simulink model "x2Stage_Rocket"  (R2022b)
settings: Solver=VariableStepAuto  StartTime=0.0  StopTime=5
model workspace: external: MATLAB File C:\Users\Trenton VerKuilen\OneDrive - lmu.edu\School\Capstone\SimscapeImportFiles\x2Stage_Rocket_DataFile.m (data not in the file)
undefined symbols (not defined in the file or in its folder): F, MIL, Moderate, sigbuilder_block, smiData, X, Y, Z
libraries: sm_lib x543, nesl_utility x11, simulink_extras x3, sharedtransform x2, dspmtrx3 x2, aerolibwind2 x2, mspsensorlib x1, aerolibatmos2 x1
(part 1 of 11)
settings Model: Creator=Poseidon  LastModifiedBy=Poseidon
settings SolverCC: MaxConsecutiveZCs=auto  ZeroCrossAlgorithm=Adaptive
settings OptimizationCC: EnhancedBackFolding=on  PassReuseOutputArgsAs=Individual arguments  ZeroExternalMemoryAtStartup=off  ZeroInternalMemoryAtStartup=off  MaxStackSize=64  OptimizeBlockOrder=speed  DifferentSizesBufferReuse=on  EfficientTunableParamExpr=on
settings DebuggingCC: IgnoredZcDiagnostic=none  ParameterTunabilityLossMsg=error
settings SFSimCC: MATLABDynamicMemAlloc=off
settings RTWCC: Description=Embedded Coder  SystemTargetFile=ert.tlc  HardwareBoard=Robot Operating System 2 (ROS 2)  TLCOptions="-aInlineSetEventsForThisBaseRateFcn=TLC_FALSE -aSuppressMultiTaskScheduler=TLC_FALSE  -aRateBasedStepFcn=0"  TemplateMakefile=ert_default_tmf  Toolchain=Colcon Tools  TargetLang=C++
settings CodeAppCC: ForceParamTrailComments=on  IgnoreCustomStorageClasses=off  OperatorAnnotations=on  SimulinkDataObjDesc=on  SFDataObjDesc=on  InsertBlockDesc=on
settings ERTTargetCC: CodeInterfacePackaging=C++ class  RootIOFormat=Structure reference

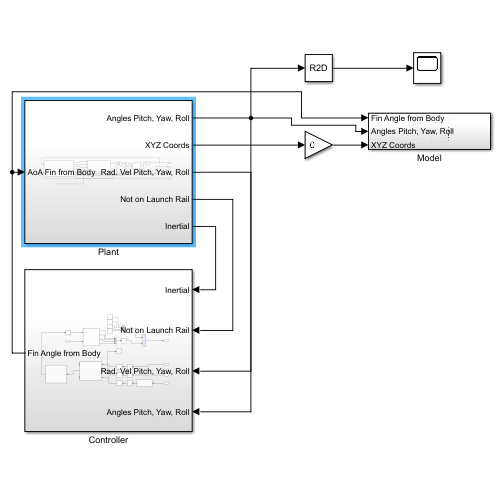
[thumbnail: Simulink's stored preview of the top-level diagram]
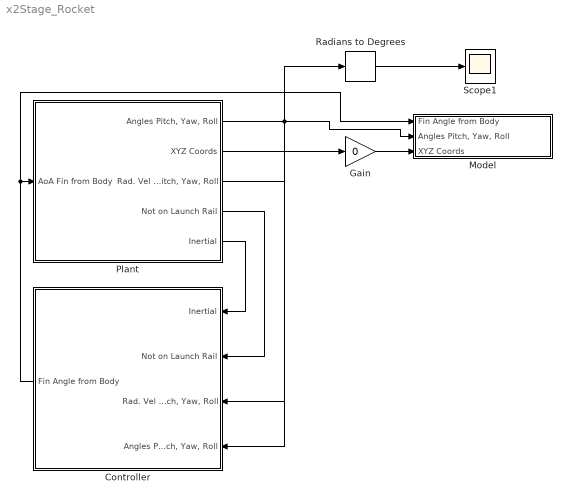
== system x2Stage_Rocket ==
  Controller : Subsystem
  Gain : Gain  Gain=0
  Model : Subsystem
  Plant : Subsystem
  Radians to Degrees : simulink_extras/Transformations/Radians to Degrees
  Scope1 : Scope
  wires:
  Radians to Degrees/1 -> Scope1/1
  Plant/3("Rad. Vel Pitch, Yaw, Roll") -> Controller/3("Rad. Vel Pitch, Yaw, Roll")
  Plant/5(Inertial) -> Controller/1(Inertial)
  Plant/4(Not on Launch Rail) -> Controller/2(Not on Launch Rail)
  Plant/2(XYZ Coords) -> Gain/1
  Gain/1 -> Model/3(XYZ Coords)
  Controller/1(Fin Angle from Body) -> Model/1(Fin Angle from Body), Plant/1(AoA Fin from Body)
  Plant/1("Angles Pitch, Yaw, Roll") -> Controller/4("Angles Pitch, Yaw, Roll"), Model/2("Angles Pitch, Yaw, Roll"), Radians to Degrees/1

== system x2Stage_Rocket/Controller ==
  Inertial : Inport
  Not on Launch Rail : Inport  Port=2
  "Rad. Vel Pitch, Yaw, Roll" : Inport  Port=3
  "Angles Pitch, Yaw, Roll" : Inport  Port=4
  Complex to Real-Imag : ComplexToRealImag  Output=Real
  Constant{,1..3} (4 alike) : Constant  Value=0
  Degrees to Radians : simulink_extras/Transformations/Degrees to Radians
  Double Click to Toggle2 : ManualSwitch  CurrentSetting=0
  MPU 6050 : mspsensorlib/IMU  DispRefFrame=NED  Temperature=25  MagneticFieldNED=[ 27.5550, -2.4169, -16.0849 ]  MagneticFieldENU=[ -2.4169, 27.5550, 16.0849 ]  SeedDouble=67  SimulateUsing=Code generation  AccelParamsMeasurementRange=160  AccelParamsResolution=0.00479  AccelParamsConstantBias=[ 0, 0, 0 ]  AccelParamsAxesMisalignment=[ 100, 0, 0; 0, 100, 0; 0, 0, 100 ]  AccelParamsNoiseDensity=[ 0, 0, 0 ]  AccelParamsBiasInstability=[ 0, 0, 0 ]  AccelParamsRandomWalk=[ 0, 0, 0 ]  AccelParamsTemperatureBias=[ 0, 0, 0 ]  AccelParamsTemperatureScaleFactor=[ 0, 0, 0 ]  GyroParamsMeasurementRange=4.36332  GyroParamsResolution=0.000133157958984  GyroParamsConstantBias=[ 0, 0, 0 ]  GyroParamsAxesMisalignment=[ 100, 0, 0; 0, 100, 0; 0, 0, 100 ]  GyroParamsAccelerationBias=[ 0, 0, 0 ]  GyroParamsNoiseDensity=[ 5.24*10^-5, 5.24*10^-5, 5.24*10^-5 ]  GyroParamsBiasInstability=[ 2.09*10^-5, 2.09*10^-5, 2.09*10^-5 ]  GyroParamsRandomWalk=[ 0, 0, 0 ]  GyroParamsTemperatureBias=[ 0, 0, 0 ]  GyroParamsTemperatureScaleFactor=[ 0, 0, 0 ]  MagParamsMeasurementRange=Inf  MagParamsResolution=0  MagParamsConstantBias=[ 0, 0, 0 ]  MagParamsAxesMisalignment=[ 100, 0, 0; 0, 100, 0; 0, 0, 100 ]  MagParamsNoiseDensity=[ 0, 0, 0 ]  MagParamsBiasInstability=[ 0, 0, 0 ]  MagParamsRandomWalk=[ 0, 0, 0 ]  MagParamsTemperatureBias=[ 0, 0, 0 ]  MagParamsTemperatureScaleFactor=[ 0, 0, 0 ]
  Mux2 : Mux
  Mux3 : Mux
  PID : Subsystem
  Rotation Angles to Quaternions : sharedtransform/Rotation Angles to Quaternions  rotationOrder=YZX  aMode=aMode
  Scope : Scope
  Transpose : Math  Operator=transpose
  Transpose1 : Math  Operator=transpose
  Transpose2 : Math  Operator=transpose
  Unscented Kalman Filter : Subsystem
  Zero-Order Hold : ZeroOrderHold  SampleTime=0.001
  Zero-Order Hold1 : ZeroOrderHold  SampleTime=0.001
  Zero-Order Hold2 : ZeroOrderHold  SampleTime=0.001
  Fin Angle from Body : Outport
  wires:
  Constant3/1 -> Mux3/4
  PID/1(Fin 1) -> Mux2/1
  Mux2/1 -> Degrees to Radians/1
  PID/4(Fin 4) -> Mux2/4
  Constant2/1 -> Mux3/3
  Constant/1 -> Mux3/1
  PID/3(Fin 3) -> Mux2/3
  PID/2(Fin 2) -> Mux2/2
  Mux3/1 -> Double Click to Toggle2/1  "Passive Fins"
  Constant1/1 -> Mux3/2
  Complex to Real-Imag/1 -> PID/1(UKF Output)
  Unscented Kalman Filter/1(Output) -> Complex to Real-Imag/1
  Degrees to Radians/1 -> Double Click to Toggle2/2  "Active Fins"
  Double Click to Toggle2/1 -> Fin Angle from Body/1
  Not on Launch Rail/1 -> PID/2(Change)
  "Rad. Vel Pitch, Yaw, Roll"/1 -> Transpose1/1
  "Angles Pitch, Yaw, Roll"/1 -> Rotation Angles to Quaternions/1
  MPU 6050/2 -> Unscented Kalman Filter/1(In2)
  Inertial/1 -> Transpose2/1
  Transpose/1 -> Zero-Order Hold2/1
  Transpose2/1 -> Zero-Order Hold/1
  Rotation Angles to Quaternions/1 -> Transpose/1
  Transpose1/1 -> Zero-Order Hold1/1
  Zero-Order Hold/1 -> MPU 6050/1
  Zero-Order Hold1/1 -> Scope/1, MPU 6050/2
  Zero-Order Hold2/1 -> MPU 6050/3
